simulink model "UDP_send_specified_control_input"  (R2023a)
settings: Solver=FixedStepAuto  StartTime=0.0  StopTime=finish_time  FixedStep=input_settings.dt  RelTol=1e-3
undefined symbols (not defined in the file): f, num_cs_sharpy, num_sensors
libraries: slrealtimeutilitieslib x2, instrumentlib x1, slrealtimeiplib x1
settings Model: Creator=ERIK  LastModifiedBy=User
settings SolverCC: AlgebraicLoopSolver=LineSearch
settings DebuggingCC: UnconnectedInputMsg=warning  UnconnectedOutputMsg=warning  UnconnectedLineMsg=warning
settings ModelReferenceCC: EnableRefExpFcnMdlSchedulingChecks=on
settings RTWCC: DLArmComputeVersion=19.05

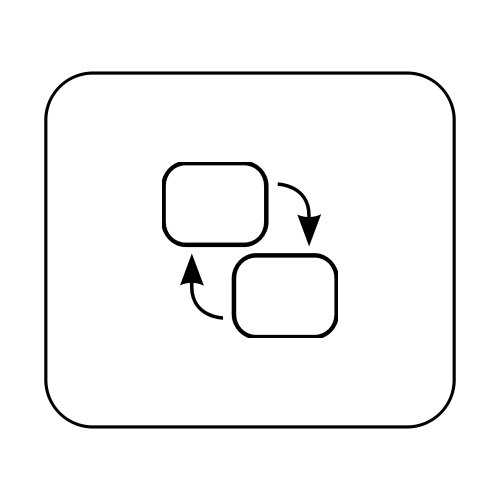
[thumbnail: Simulink's stored preview of the top-level diagram]
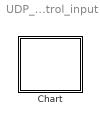
== system UDP_send_specified_control_input ==
  Chart : Stateflow chart  TreatAsAtomicUnit=on

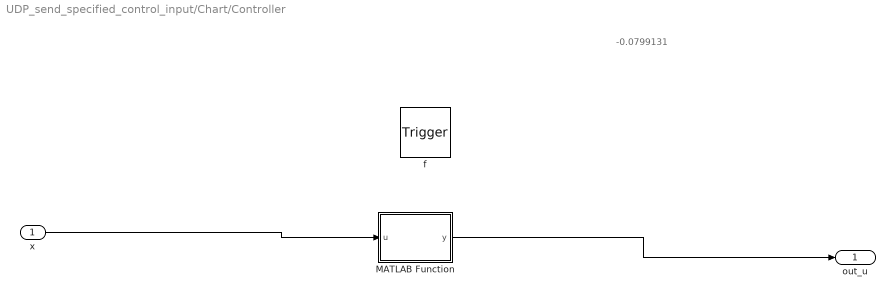
== system UDP_send_specified_control_input/Chart/Controller ==
  note: -0.0799131
  x : Inport  OutDataTypeStr=double  PortDimensions=num_sensors
  f : TriggerPort  TriggerType=function-call  VariantControl=(inherit)
      settings: CopyFcn=Stateflow.SLINSF.SimulinkMan.removeBlockPreDeleteFcn  PreDeleteFcn=Stateflow.SLINSF.SimulinkMan.unsafePredeleteFcn
  MATLAB Function : MATLAB Function  TreatAsAtomicUnit=on
  out_u : Outport
  wires:
  MATLAB Function/1(y) -> out_u/1
  x/1 -> MATLAB Function/1(u)

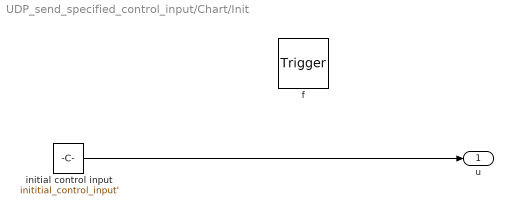
== system UDP_send_specified_control_input/Chart/Init ==
  f : TriggerPort  TriggerType=function-call  VariantControl=(inherit)
      settings: CopyFcn=Stateflow.SLINSF.SimulinkMan.removeBlockPreDeleteFcn  PreDeleteFcn=Stateflow.SLINSF.SimulinkMan.unsafePredeleteFcn
  initial control input : Constant  Value=inititial_control_input'
  u : Outport
  wires:
  initial control input/1 -> u/1

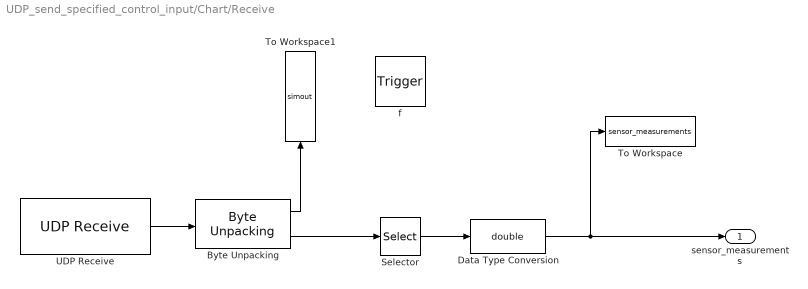
== system UDP_send_specified_control_input/Chart/Receive ==
  f : TriggerPort  TriggerType=function-call  VariantControl=(inherit)
      settings: CopyFcn=Stateflow.SLINSF.SimulinkMan.removeBlockPreDeleteFcn  PreDeleteFcn=Stateflow.SLINSF.SimulinkMan.unsafePredeleteFcn
  "Byte Unpacking " : slrealtimeutilitieslib/Byte Unpacking  MaskUnpackedDataTypes={'uint8' 'single'}  MaskUnpackedDataSizes={5 num_sensors*2}  MaskAlignment=1
  Data Type Conversion : DataTypeConversion  OutDataTypeStr=double  SaturateOnIntegerOverflow=off  RndMeth=Floor
  Selector : Selector  InputPortWidth=num_sensors*2  IndexOptions=Index vector (dialog)  Indices=2:2:2*num_sensors  OutputSizes=1
  To Workspace : ToWorkspace  VariableName=sensor_measurements  SaveFormat=Timeseries  SampleTime=-1
  To Workspace1 : ToWorkspace  VariableName=simout  SaveFormat=Timeseries  SampleTime=-1
  UDP Receive : instrumentlib/UDP Receive  LocalAddress=127.0.0.1  LocalPort=59006  EnablePortSharing=off  Host=127.0.0.1  Port=59016  GetLatestData=on  DataSize=149  DataType=uint8  ASCIIFormatting=%f,  Terminator=LF  CustomTerminator=10  ByteOrder=little-endian  EnableBlockingMode=on  Timeout=600  SampleTime=-1  SimulateUsing=Interpreted execution
  sensor_measurements : Outport
  wires:
  UDP Receive/1 -> "Byte Unpacking "/1
  Selector/1 -> Data Type Conversion/1
  Data Type Conversion/1 -> To Workspace/1, sensor_measurements/1
  "Byte Unpacking "/2 -> Selector/1
  "Byte Unpacking "/1 -> To Workspace1/1

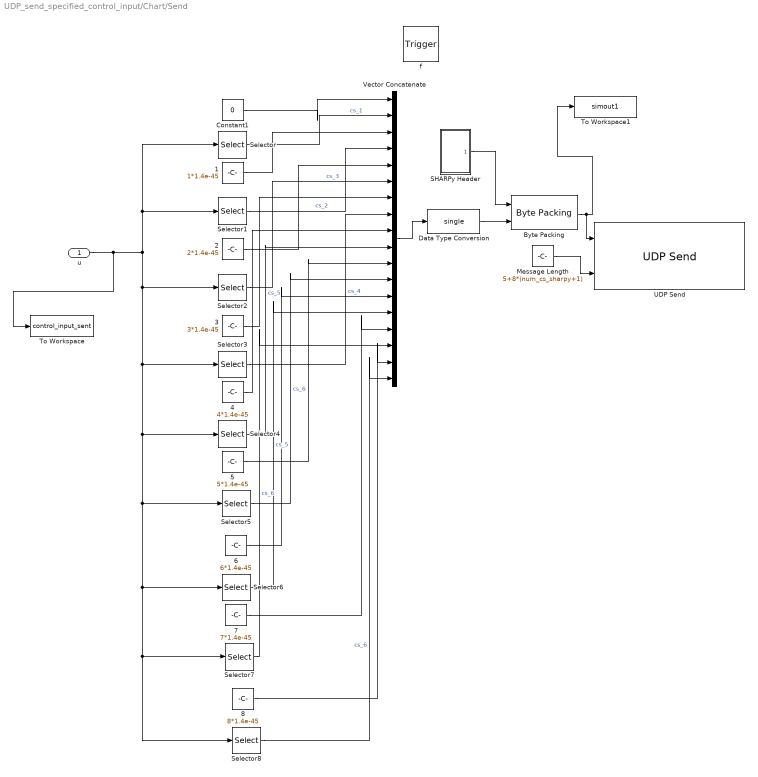
== system UDP_send_specified_control_input/Chart/Send ==
  u : Inport  OutDataTypeStr=double  PortDimensions=num_cs_sharpy+1
  f : TriggerPort  TriggerType=function-call  VariantControl=(inherit)
      settings: CopyFcn=Stateflow.SLINSF.SimulinkMan.removeBlockPreDeleteFcn  PreDeleteFcn=Stateflow.SLINSF.SimulinkMan.unsafePredeleteFcn
  1 : Constant  Value=1*1.4e-45
  2 : Constant  Value=2*1.4e-45
  3 : Constant  Value=3*1.4e-45
  4 : Constant  Value=4*1.4e-45
  5 : Constant  Value=5*1.4e-45
  6 : Constant  Value=6*1.4e-45
  7 : Constant  Value=7*1.4e-45
  8 : Constant  Value=8*1.4e-45
  "Byte Packing " : slrealtimeutilitieslib/Byte Packing  MaskPackedDataType=uint8  MaskUnpackedDataTypes={'uint8' 'single'}  MaskAlignment=1
  Constant1 : Constant  Value=0
  Data Type Conversion : DataTypeConversion  OutDataTypeStr=single  SaturateOnIntegerOverflow=off  RndMeth=Floor
  Message Length : Constant  Value=5+8*(num_cs_sharpy+1)
  SHARPy Header : Subsystem
  Selector : Selector  InputPortWidth=num_cs_sharpy+1  IndexOptions=Index vector (dialog)  Indices=[1]  OutputSizes=1
  Selector1 : Selector  InputPortWidth=num_cs_sharpy+1  IndexOptions=Index vector (dialog)  Indices=[2]  OutputSizes=1
  Selector2 : Selector  InputPortWidth=num_cs_sharpy+1  IndexOptions=Index vector (dialog)  Indices=[3]  OutputSizes=1
  Selector3 : Selector  InputPortWidth=num_cs_sharpy+1  IndexOptions=Index vector (dialog)  Indices=[4]  OutputSizes=1
  Selector4 : Selector  InputPortWidth=num_cs_sharpy+1  IndexOptions=Index vector (dialog)  Indices=[5]  OutputSizes=1
  Selector5 : Selector  InputPortWidth=num_cs_sharpy+1  IndexOptions=Index vector (dialog)  Indices=[6]  OutputSizes=1
  Selector6 : Selector  InputPortWidth=num_cs_sharpy+1  IndexOptions=Index vector (dialog)  Indices=[7]  OutputSizes=1
  Selector7 : Selector  InputPortWidth=num_cs_sharpy+1  IndexOptions=Index vector (dialog)  Indices=[8]  OutputSizes=1
  Selector8 : Selector  InputPortWidth=num_cs_sharpy+1  IndexOptions=Index vector (dialog)  Indices=[9]  OutputSizes=1
  To Workspace : ToWorkspace  VariableName=control_input_sent  SaveFormat=Timeseries  SampleTime=-1
  To Workspace1 : ToWorkspace  VariableName=simout1  SaveFormat=Timeseries  SampleTime=-1
  UDP Send : slrealtimeiplib/UDP Send  useHostTargetConn=on  toAddress=127.0.0.1  toPort=64016  sampleTime=-1  enableMessage=off  localPort=59001
  Vector Concatenate : Concatenate  NumInputs=18
  wires:
  u/1 -> To Workspace/1, Selector/1, Selector1/1, Selector8/1, Selector7/1, Selector6/1, Selector5/1, Selector4/1, Selector3/1, Selector2/1
  Selector/1 -> Vector Concatenate/2  "cs_1"
  Constant1/1 -> Vector Concatenate/1
  Data Type Conversion/1 -> "Byte Packing "/2
  "Byte Packing "/1 -> To Workspace1/1, UDP Send/1
  Message Length/1 -> UDP Send/2
  SHARPy Header/1(Header) -> "Byte Packing "/1
  Selector1/1 -> Vector Concatenate/4  "cs_2"
  Selector2/1 -> Vector Concatenate/6  "cs_3"
  Selector3/1 -> Vector Concatenate/8  "cs_4"
  1/1 -> Vector Concatenate/3
  2/1 -> Vector Concatenate/5
  3/1 -> Vector Concatenate/7
  Vector Concatenate/1 -> Data Type Conversion/1
  4/1 -> Vector Concatenate/9
  Selector4/1 -> Vector Concatenate/10  "cs_5"
  5/1 -> Vector Concatenate/11
  Selector5/1 -> Vector Concatenate/12  "cs_6"
  6/1 -> Vector Concatenate/13
  Selector6/1 -> Vector Concatenate/14  "cs_5"
  7/1 -> Vector Concatenate/15
  Selector7/1 -> Vector Concatenate/16  "cs_6"
  8/1 -> Vector Concatenate/17
  Selector8/1 -> Vector Concatenate/18  "cs_6"

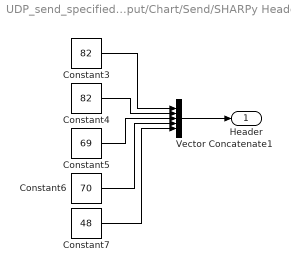
== system UDP_send_specified_control_input/Chart/Send/SHARPy Header ==
  Constant3 : Constant  Value=82  OutDataTypeStr=uint8
  Constant4 : Constant  Value=82  OutDataTypeStr=uint8
  Constant5 : Constant  Value=69  OutDataTypeStr=uint8
  Constant6 : Constant  Value=70  OutDataTypeStr=uint8
  Constant7 : Constant  Value=48  OutDataTypeStr=uint8
  Vector Concatenate1 : Concatenate  NumInputs=5
  Header : Outport
  wires:
  Constant7/1 -> Vector Concatenate1/5
  Constant5/1 -> Vector Concatenate1/3
  Constant6/1 -> Vector Concatenate1/4
  Constant4/1 -> Vector Concatenate1/2
  Constant3/1 -> Vector Concatenate1/1
  Vector Concatenate1/1 -> Header/1

== matlab function UDP_send_specified_control_input/Chart/Controller/MATLAB Function ==
  data: u input; y output
function y = fcn(u)

y = [0.008172 0.008172 0.008172  0.008172 0.008172  0.008172 0.008172 0.008172 -0.565215]';

== stateflow chart UDP_send_specified_control_input/Chart ==
  state u=Init [function]
  state Send(u) [function]
  state Stateflow
    entry:  u=Init();
    during: Send(u);
    x =Receive();
    u = Controller(x);
  state sensor_measurements = Receive [function]
  state out_u = Controller(x) [function]
  (default) -> Stateflow
  data: u function_output; u function_input double size=num_cs_sharpy+1; sensor_measurements function_output; out_u function_output; x function_input double size=num_sensors; x local; u local
